simulink model "classprojectfinal"  (R2023b)
settings: Solver=FixedStepDiscrete  StartTime=0.0  StopTime=75  FixedStep=0.025  RelTol=1e-3
settings Model: Creator=farid  LastModifiedBy=nita9
settings OptimizationCC: ReuseModelBlockBuffer=off

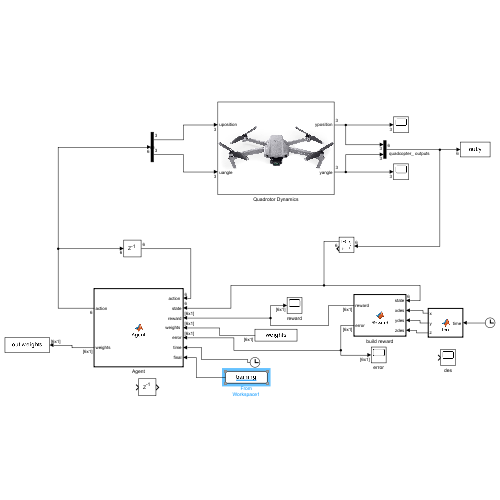
[thumbnail: Simulink's stored preview of the top-level diagram]
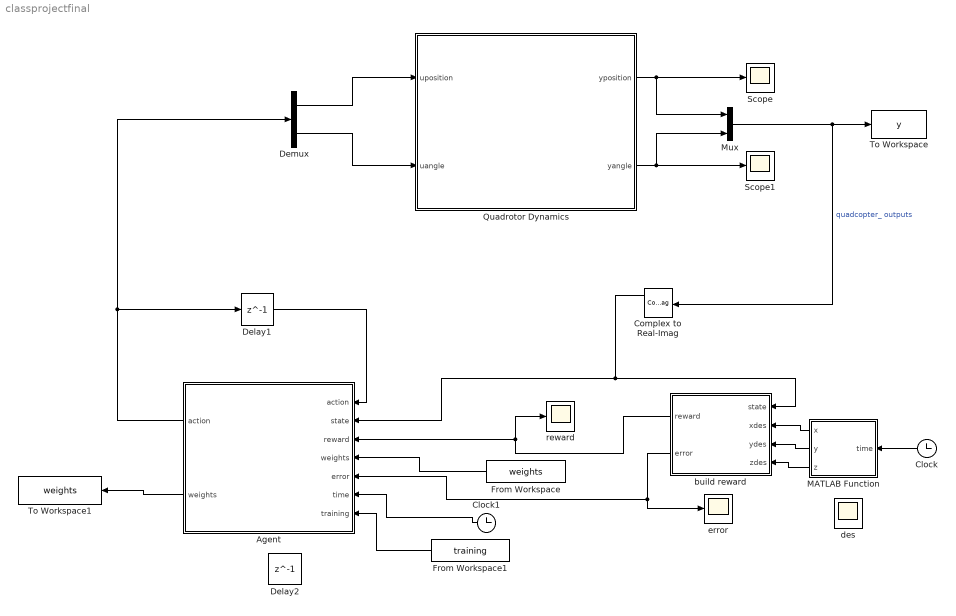
== system classprojectfinal ==
  Agent : MATLAB Function  TreatAsAtomicUnit=on
  Clock : Clock
  Clock1 : Clock
  Complex to Real-Imag : ComplexToRealImag
  Delay1 : Delay  DelayLength=1  InitialCondition=0
  Delay2 : Delay  DelayLength=1  InitialCondition=0
  Demux : Demux  Outputs=2
      settings: DisplayOption=none
  From Workspace : FromWorkspace  VariableName=weights  SampleTime=-1
  From Workspace1 : FromWorkspace  VariableName=training  SampleTime=-1
  MATLAB Function : MATLAB Function  TreatAsAtomicUnit=on
  Mux : Mux  Inputs=2
  Quadrotor Dynamics : Subsystem
      mask Display: image('$imagefile'); % Use "Edit Image" on toolstrip to change.
  Scope : Scope
  Scope1 : Scope
  To Workspace : ToWorkspace  VariableName=y  SampleTime=-1
      settings: MaxDataPoints=Inf
  To Workspace1 : ToWorkspace  VariableName=weights  SaveFormat=Timeseries  SampleTime=-1
  build reward : MATLAB Function  TreatAsAtomicUnit=on
  des : Scope
  error : Scope
  reward : Scope
  wires:
  Mux/1 -> Complex to Real-Imag/1, To Workspace/1  "quadcopter_ outputs"
  Quadrotor Dynamics/2(yangle) -> Mux/2, Scope1/1
  Quadrotor Dynamics/1(yposition) -> Scope/1, Mux/1
  Demux/2 -> Quadrotor Dynamics/2(uangle)
  Demux/1 -> Quadrotor Dynamics/1(uposition)
  build reward/1(reward) -> reward/1, Agent/3(reward)
  Agent/2(weights) -> To Workspace1/1
  From Workspace/1 -> Agent/4("weights ")
  Delay1/1 -> Agent/1("action ")
  build reward/2(error) -> error/1, Agent/5(error)
  Complex to Real-Imag/1 -> build reward/1(state), Agent/2(state)
  MATLAB Function/1(x) -> build reward/2(xdes)
  Clock/1 -> MATLAB Function/1(time)
  MATLAB Function/2(y) -> build reward/3(ydes)
  MATLAB Function/3(z) -> build reward/4(zdes)
  Agent/1(action) -> Delay1/1, Demux/1
  Clock1/1 -> Agent/6(time)
  From Workspace1/1 -> Agent/7(training)

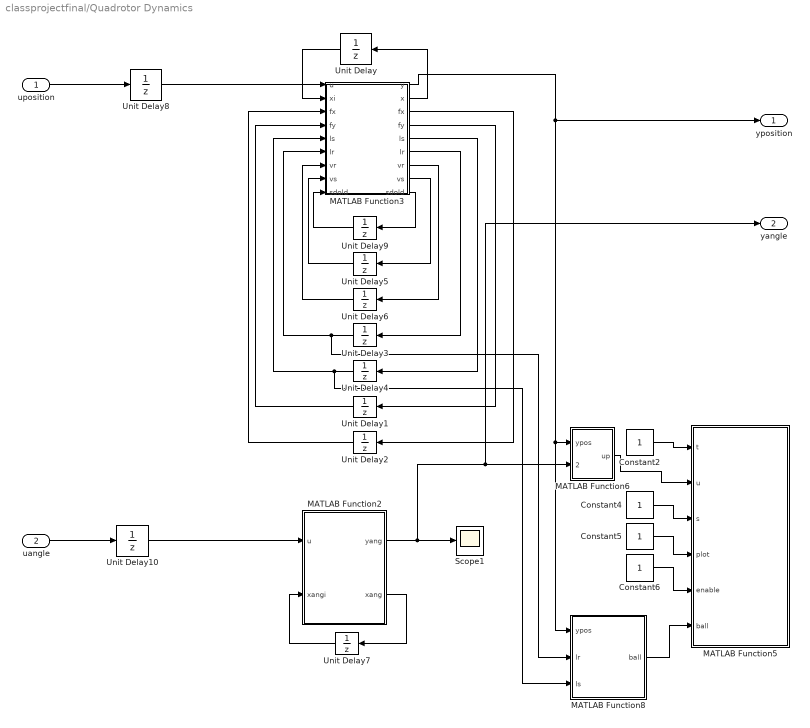
== system classprojectfinal/Quadrotor Dynamics ==
  uposition : Inport
  uangle : Inport  Port=2
  Constant{2,4..6} (4 alike) : Constant
  MATLAB Function2 : MATLAB Function  TreatAsAtomicUnit=on
  MATLAB Function3 : MATLAB Function  TreatAsAtomicUnit=on
  MATLAB Function5 : MATLAB Function  TreatAsAtomicUnit=on
  MATLAB Function6 : MATLAB Function  TreatAsAtomicUnit=on
  MATLAB Function8 : MATLAB Function  TreatAsAtomicUnit=on
  Scope1 : Scope
  Unit Delay : UnitDelay  InitialCondition=|  SampleTime=-1  HasFrameUpgradeWarning=on
      | [0
      | 0
      | 0
      | 0
      | 1.50000000000000
      | 0]
  Unit Delay{1..6,9} (7 alike) : UnitDelay  SampleTime=-1  HasFrameUpgradeWarning=on
  Unit Delay10 : UnitDelay  InitialCondition=|  SampleTime=-1  HasFrameUpgradeWarning=on
      | [0
      | 0
      | 0]
  Unit Delay7 : UnitDelay  InitialCondition=|  SampleTime=-1  HasFrameUpgradeWarning=on
      | [0
      | 0
      | 0
      | 0
      | 0
      | 0]
  Unit Delay8 : UnitDelay  InitialCondition=|  SampleTime=-1  HasFrameUpgradeWarning=on
      | [0
      | 0
      | 0]
  yposition : Outport
  yangle : Outport  Port=2
  wires:
  Unit Delay6/1 -> MATLAB Function3/7("vr ")
  MATLAB Function3/2(x) -> Unit Delay/1
  MATLAB Function3/5(ls) -> Unit Delay4/1
  MATLAB Function2/1(yang) -> Scope1/1, yangle/1, MATLAB Function6/2(yang)
  Constant4/1 -> MATLAB Function5/3(s)
  Constant2/1 -> MATLAB Function5/1(t)
  MATLAB Function3/4(fy) -> Unit Delay1/1
  Unit Delay/1 -> MATLAB Function3/2(xi)
  MATLAB Function3/9(sdold) -> Unit Delay9/1
  MATLAB Function8/1(ball) -> MATLAB Function5/6(ball)
  Unit Delay4/1 -> MATLAB Function8/3(ls), MATLAB Function3/5("ls ")
  Unit Delay2/1 -> MATLAB Function3/3("fx ")
  MATLAB Function2/2(xang) -> Unit Delay7/1
  MATLAB Function3/1(y) -> yposition/1, MATLAB Function8/1(ypos), MATLAB Function6/1(ypos)
  MATLAB Function3/6(lr) -> Unit Delay3/1
  Constant5/1 -> MATLAB Function5/4(plot)
  MATLAB Function3/8(vs) -> Unit Delay5/1
  Unit Delay3/1 -> MATLAB Function8/2(lr), MATLAB Function3/6("lr ")
  Unit Delay5/1 -> MATLAB Function3/8("vs ")
  Constant6/1 -> MATLAB Function5/5(enable)
  MATLAB Function6/1(up) -> MATLAB Function5/2(u)
  Unit Delay7/1 -> MATLAB Function2/2(xangi)
  MATLAB Function3/7(vr) -> Unit Delay6/1
  MATLAB Function3/3(fx) -> Unit Delay2/1
  Unit Delay9/1 -> MATLAB Function3/9("sdold ")
  Unit Delay1/1 -> MATLAB Function3/4("fy ")
  uposition/1 -> Unit Delay8/1
  uangle/1 -> Unit Delay10/1
  Unit Delay8/1 -> MATLAB Function3/1(u)
  Unit Delay10/1 -> MATLAB Function2/1(u)

== matlab function classprojectfinal/Quadrotor Dynamics/MATLAB Function5 ==
  data: t input; u input; s input; plot input; enable input; ball input
function qd_plot(t,u,s, plot, enable,ball)
    quad.nrotors =4;
    quad.d = 0.17;
    quad.r = 0.1;
    
    a1s = zeros(1, quad.nrotors);
    b1s = zeros(1, quad.nrotors);

    
    % vehicle dimensons
    d = quad.d; %Hub displacement from COG
    r = quad.r; %Rotor radius
    D = zeros(3,4);
    C = zeros(3,4);
    for i = 1:quad.nrotors
        theta = (i-1)/quad.nrotors*2*pi;
        %   Di      Rotor hub displacements (1x3)
        % first rotor is on the x-axis, clockwise order looking down from above
        D(:,i) = [ d*cos(theta); d*sin(theta); 0];
%         scal = s(1)/4;
        scal = 0.2/4;
        %Attitude center displacements
        C(:,i) = [ scal*cos(theta); scal*sin(theta); 0];
    end
    
    if enable == 1
        %draw ground
        figure(1);
        clf;
        if length(s) == 1
            axis([-0.5 1.5 -0.5 1.5 0 2]);
        else
%             axis([-s(1) s(1) -s(1) s(1) 0 s(2)])
            axis([-0.5 s(1) -0.5 s(1) 0 s(2)])
            s = 1.5;
        end
        hold on;
        
        % plot the ground boundaries and the big cross
        plot3([-0.5 -0.5],[-0.5 1],[0 0],'-b')
        plot3([-0.5 1.5],[-0.5 -0.5],[0 0],'-b')
        plot3([-0.5 1.5],[-0.5 1.5],[0 0],'-b')
        plot3([1.5 -0.5],[1.5 1.5],[0 0],'-b')
        plot3([1.5 1.5],[1.5 -0.5],[0 0],'-b')
        plot3([-0.5 1.5],[1.5 -0.5],[0 0],'-b')
        
        plot3([0 1], [0 0], [1.5 1.5],':r','LineWidth',0.2)
        plot3([1 1], [0 1], [1.5 1.5],':r','LineWidth',0.2)
        plot3([0 1], [1 1], [1.5 1.5],':r','LineWidth',0.2)
        plot3([0 0], [0 1], [1.5 1.5],':r','LineWidth',0.2)
        
        plot3([0 1], [0 0], [1 1],':r','LineWidth',0.2)
        plot3([1 1], [0 1], [1 1],':r','LineWidth',0.2)
        plot3([0 1], [1 1], [1 1],':r','LineWidth',0.2)
        plot3([0 0], [0 1], [1 1],':r','LineWidth',0.2)
        %READ STATE
        z = [u(1);u(2);u(3)];
        n = [u(4);u(5);u(6)];
        
        %PREPROCESS ROTATION MATRIX
        phi = n(1);    %Euler angles
        the = n(2);
        psi = n(3);
        
        R = [cos(the)*cos(phi) sin(psi)*sin(the)*cos(phi)-cos(psi)*sin(phi) cos(psi)*sin(the)*cos(phi)+sin(psi)*sin(phi);   %BBF > Inertial rotation matrix
            cos(the)*sin(phi) sin(psi)*sin(the)*sin(phi)+cos(psi)*cos(phi) cos(psi)*sin(the)*sin(phi)-sin(psi)*cos(phi);
            -sin(the)         sin(psi)*cos(the)                            cos(psi)*cos(the)];
        
        %Manual Construction
        %Q3 = [cos(psi) -sin(psi) 0;sin(psi) cos(psi) 0;0 0 1];   %Rotation mappings
        %Q2 = [cos(the) 0 sin(the);0 1 0;-sin(the) 0 cos(the)];
        %Q1 = [1 0 0;0 cos(phi) -sin(phi);0 sin(phi) cos(phi)];
        %R = Q3*Q2*Q1;    %Rotation matrix
        
        %CALCULATE FLYER TIP POSITONS USING COORDINATE FRAME ROTATION
        F = [1 0 0;0 -1 0;0 0 -1];
        
        %Draw flyer rotors
        t = [0:pi/8:2*pi];
        circle = zeros(3,17);
        for j = 1:length(t)
            circle(:,j) = [r*sin(t(j));r*cos(t(j));0];
        end
        hub = zeros(3,4);
        tippath = zeros(3,17,4);
        for i = 1:quad.nrotors
            hub(:,i) = F*(z + R*D(:,i)); %points in the inertial frame
            center = F*z;
            ball_pos = F*ball;
            plot3(center(1),center(2),center(3),'r.')
            plot3(ball_pos(1),ball_pos(2),ball_pos(3),'co')
            plot3([center(1) ball_pos(1)],[center(2) ball_pos(2)],[center(3) ball_pos(3)],'-b')
            
            q = 1; %Flapping angle scaling for output display - makes it easier to see what flapping is occurring
            Rr = [cos(q*a1s(i))  sin(q*b1s(i))*sin(q*a1s(i)) cos(q*b1s(i))*sin(q*a1s(i));   %Rotor > Plot frame
                0              cos(q*b1s(i))               -sin(q*b1s(i));
                -sin(q*a1s(i)) sin(q*b1s(i))*cos(q*a1s(i)) cos(q*b1s(i))*cos(q*a1s(i))];
            
            tippath(:,:,i) = F*R*Rr*circle;
            plot3([hub(1,i)+tippath(1,:,i)],[hub(2,i)+tippath(2,:,i)],[hub(3,i)+tippath(3,:,i)],'b-')
        end
        
        %Draw flyer
        hub0 = F*z;  % centre of vehicle
        for i = 1:quad.nrotors
            % line from hub to centre plot3([hub(1,N) hub(1,S)],[hub(2,N) hub(2,S)],[hub(3,N) hub(3,S)],'-b')
            plot3([hub(1,i) hub0(1)],[hub(2,i) hub0(2)],[hub(3,i) hub0(3)],'-b')
            
            % plot a circle at the hub itself
            plot3([hub(1,i)],[hub(2,i)],[hub(3,i)],'o')
        end
        
        % plot the vehicle's centroid on the ground plane
        plot3([z(1) 0],[-z(2) 0],[0 0],'--k')
        plot3([z(1)],[-z(2)],[0],'xk')
        plot3([z(1) z(1)],[-z(2) -s],[0 0],'r-.')

        % label the axes
        xlabel('x');
        ylabel('y');
        zlabel('z (height above ground)');
        view([-5 -2 5]);
    end;

== matlab function classprojectfinal/Quadrotor Dynamics/MATLAB Function6 ==
  data: up output; ypos input; yang input
function up= upp(ypos,yang)
up = [ypos(1) -ypos(2) -ypos(3) yang(1) yang(2) yang(3)];

== matlab function classprojectfinal/Quadrotor Dynamics/MATLAB Function8 ==
  data: ball output; ypos input; lr input; ls input
function ball= balll(ypos,lr,ls)
ball=[ypos(1)+lr(1) -(ypos(2)+ls(1)) 1-ypos(3)-sqrt(abs(0.25-lr(1)^2-ls(1)^2))]';

== matlab function classprojectfinal/Agent ==
  data: action input; state input size=6; reward input; weights input; error input; action output; weights output size=size(State); time input; training input
function [action, weights] = Agent(action, state, reward, weights, error, time, training)
%%

% 
% alpha = 0.011;
L = 1.5; 
w = 0.5;
gamma = L / w; 

%
if(training == 0) % training

    if(time > 5)

        alpha = 0.015;
        exploration_variance = 0.05 * gamma;
        noise = exploration_variance * randn(size(state));
        state = state + noise;

    else

        alpha = 0.01;
        exploration_variance = 1 * gamma;
        noise = exploration_variance * randn(size(state));
        state = state + noise;

    end

else % not training

    alpha = 0.15;
    exploration_variance = 0;
    noise = exploration_variance * randn(size(state));
    state = state + noise;

end

% old version
activation = state ./ gamma + error + action;
Q_last = weights .* (activation); 

% 
max_action = 0.0627;
action = max_action .* Q_last; 

% 
for i = 1:6

    weights(i) = weights(i) + alpha * reward(i) * activation(i);  

end

end

%% OLD VERSION

% % Parameters
% alpha = 0.01;
% gamma = 0.1;
% 
% % Initialize weights if not provided
% weights = zeros(size(weights_last));
% if isempty(weights_last)
%     weights_last = 0.1 * randn(size(state));  % Random initialization
% else
%     weights_last = weights_last;  % Use last weight if provided
% end
% 
% % old version
% activation = state + error + action;
% action = weights_last .* (activation);  
% 
% % Adding noise for exploration: Gaussian noise
% % exploration_variance = 0.05; % Adjust as necessary for adequate exploration
% % noise = exploration_variance * randn(size(action));  % Same dimension as action
% % action = action + noise;
% 
% % Ensure actions are within bounds
% max_action = 0.0627;
% action_scaling_factor = 0.6;  % Reduce this value to scale down actions
% action = action_scaling_factor * max(min(action, max_action), -max_action);  % Clipping each element
% 
% % Assuming RewardVector is [6 x 1], compatible with State [6 x 1]
% % Simple policy gradient update using element-wise multiplication
% gradients = state .* reward;  % Element-wise product for gradient calculation
% weights_last = weights_last + alpha * gradients;  % Update weights element-wise
% 
% % Return the new weights and the action
% end

%% BROKEN VERSION

% function [action, weights_last, Q] = Agent(action, state, reward, weights_last, error, Q_last)

% %
% weights = [0; 0; 0; 0; 0; 0];
% alpha = 0.01;
% gamma = 0.01;
% actions_x = [-0.067, -0.03, 0.0, 0.03, 0.067];
% actions_y = [-0.067, -0.03, 0.0, 0.03, 0.067];
% actions_z = [-0.067, -0.03, 0.0, 0.03, 0.067];
% actions_alpha = [-0.0777, -0.03, 0.0, 0.03, 0.0777];
% actions_beta = [-0.0777, -0.03, 0.0, 0.03, 0.0777];
% actions_gamma = [-0.0777, -0.03, 0.0, 0.03, 0.0777];
% actions = [actions_x; actions_y; actions_z; actions_alpha; actions_beta; actions_gamma];
% 
% %
% Q_best = -10^6;
% idx = zeros(6, 1);
% for i = 1:5 % x
%     for j = 1:5 % y
%         for k = 1:5 % z
%             for l = 1:5 % phi
%                 for m = 1:5 % theta
%                     for n = 1:5 % psi
% 
%                         %
%                         Q_current = weights_last(1) * (state(1) + actions_x(i) + error(1)) + ...
%                                     weights_last(2) * (state(2) + actions_y(j) + error(2)) + ...
%                                     weights_last(3) * (state(3) + actions_z(k) + error(3)) + ...
%                                     weights_last(4) * (state(4) + actions_alpha(l) + error(4)) + ...
%                                     weights_last(5) * (state(5) + actions_beta(m) + error(5)) + ...
%                                     weights_last(6) * (state(6) + actions_gamma(n) + error(6));
% 
%                         %
%                         if(Q_current > Q_best)
% 
%                             Q_best = Q_current;
%                             idx = [i; j; k; l; m; n];
% 
%                         end
% 
%                     end
%                 end
%             end
%         end
%     end
% end
% 
% %
% % difference= Reward + gamma*Qmax - Q_tminus; %% or should it be weights_tminus
% % weights = weights_last;
% for i = 1:6
% 
%     action(i) = actions(i, idx(i));
%     diff = (reward(i) + gamma * Q_best) - Q_last;
%     Q_best = Q_best + alpha * diff;
%     weights_last(i) = weights_last(i) + alpha * diff * (state(i) + action(i) + error(i));
% 
%     if(abs(weights_last(i)) > 0.02)
% 
%         weights_last(i) = sign(weights_last(i)) * 0.02;
% 
%     end
% 
% end
% 
% %
% % action = [actions{1}(action_indexes(1)); actions{2}(action_indexes(2)); actions{3}(action_indexes(3)); actions{4}(action_indexes(4)); actions{5}(action_indexes(5)); actions{6}(action_indexes(6))];
% % weights = weights_last;
% Q = Q_best;
% 
% end

%%

== matlab function classprojectfinal/build reward ==
  data: state input; xdes input; reward output; error output; ydes input; zdes input
function [reward, error] = Reward(state, xdes, ydes, zdes)

%
error = zeros(6, 1);
error = [3 * (state(1) - xdes); -6 * (state(2) - ydes); -3 * (state(3) - zdes); -3 * state(4); -3 * state(5); -3 * state(6)];

% Squared position error (assuming target is provided correctly)
R_position = [30 * (state(1)-xdes)^2 ; 30 * (state(2)-ydes)^2; 30 * (state(3)-zdes)^2];

% Angle error penalization (assuming perfect angles are 0)
R_angle = 30 .* [(state(4))^2; (state(5))^2; (state(6))^2];

%
reward = zeros(6, 1);
reward = [-R_position; -R_angle];

== matlab function classprojectfinal/MATLAB Function ==
  data: time input; x output; y output; z output
function [x, y, z] = fcn(time)

%
if(time == 0)

    des = [0; 0; 1.5];

else

    ref = load("squaretrajectory.mat");
    idx = time / 0.025;
    des = ref.ref(:, idx);

end

x = des(1);
y = des(2);
z = des(3);

== matlab function classprojectfinal/Quadrotor Dynamics/MATLAB Function2 ==
  data: yang output; xang output; u input; xangi input
function [yang,xang]= sysang(u,xangi)
Ts = 1/40;
g = 9.81;
A = [1,0.0250000000000000,0,0,0,0;0,1,0,0,0,0;0,0,1,0.0250000000000000,0,0;0,0,0,1,0,0;0,0,0,0,1,0.0250000000000000;0,0,0,0,0,1];
B = [0.0416666666666667,0,0;3.33333333333333,0,0;0,0.0416666666666667,0;0,3.33333333333333,0;0,0,0.0240384615384615;0,0,1.92307692307692];
C = [1,0,0,0,0,0;0,0,1,0,0,0;0,0,0,0,1,0];
D = zeros(3,3);
xang = zeros(6,1);
yang = zeros(3,1);
xang = A*xangi + B*u;
yang = C*xang + D*u;

== matlab function classprojectfinal/Quadrotor Dynamics/MATLAB Function3 ==
  data: y output; x output; u input; xi input; fx input; fy input; fx output; fy output; ls input; lr input; ls output; lr output; vr input; vs input; vr output; vs output; sdold input; sdold output
function [y,x, fx,fy,ls,lr,vr,vs,sdold]= syspos(u,xi,fx,fy,ls,lr,vr,vs,sdold)
Ts = 1/40;
g = 9.81;
A = [1 0.025 0 0 0 0;0 1 0 0 0 0;0 0 1 0.025 0 0;0 0 0 1 0 0;0 0 0 0 1 0.025;0 0 0 0 0 1];
B = [-0.003065625 0 0;-0.24525 0 0;0 0.003065625 0;0 0.24525 0;0 0 0.0003125;0 0 0.025];
C = [1 0 0 0 0 0;0 0 1 0 0 0;0 0 0 0 1 0];
D = zeros(3,3);
x = zeros(6,1);
y = zeros(3,1);
x = A*xi + B*u;
y = C*x + D*u;
x(2) = x(2) - fx;
x(4) = x(4) - fy;


xdold = x(2)-xi(2);
ydold = x(4)-xi(4);
zdold = x(6)-xi(6);

% sqrt(complex(x))
yita = sqrt(abs(0.5^2-lr^2-ls^2));
vrold = vr;
vsold = vs;
vr = ( yita^4*xdold - lr*yita^3*zdold + lr*ls*yita^2*sdold +...
    (lr*0.5^2-lr*ls^2)*vr^2 +...
    (lr*0.5^2-lr^3)*vs^2 +...
    2*vr*vs*lr^2*ls + lr*g*yita^3 )/((ls^2-0.5^2)*yita^2);
lr = lr + vr*Ts;
rdold = vr-vrold;

vs = ( yita^4*ydold - ls*yita^3*zdold + lr*ls*yita^2*rdold +...
    (ls*0.5^2-ls*lr^2)*vs^2 +...
    (ls*0.5^2-ls^3)*vr^2 +...
    2*vr*vs*ls^2*lr + ls*g*yita^3 )/((lr^2-0.5^2)*yita^2);
ls = ls + vs*Ts;
% sdold = vs(1,i+1);
sdold = vs(1)-vsold(1);

fx = 0.3*(xdold+rdold);
fy = 0.3*(ydold+sdold);
